simulink model "EMD_model_3"  (R2018b)
settings: Solver=ode45  StartTime=0  StopTime=setStopTime  FixedStep=0.0005  RelTol=1e-3  EnableMultiTasking=on
model workspace (MAT data in the model file):
  Body = timeseries
  Body.Name = 'unnamed'
  Body.DataInfo = tsdata.datametadata
  Body.DataInfo.Interpolation = tsdata.interpolation
  Body.DataInfo.Interpolation.Fhandle : function handle (value not decoded)
  Body.DataInfo.Interpolation.Name = 'linear'
  Body.TimeInfo = tsdata.timemetadata
  Body.TimeInfo.Length = 1
  Body.TimeInfo.DuplicateTimes = 0
  Body.TimeInfo.Time_ = 0
  Body.TimeInfo.Initialized = 1
  Body.QualityInfo = tsdata.qualmetadata
  Body.Data_ = 0
  Head = timeseries
  Head.Name = 'unnamed'
  Head.DataInfo = tsdata.datametadata
  Head.DataInfo.Interpolation = tsdata.interpolation
  Head.DataInfo.Interpolation.Fhandle : function handle (value not decoded)
  Head.DataInfo.Interpolation.Name = 'linear'
  Head.TimeInfo = tsdata.timemetadata
  Head.TimeInfo.Length = 1
  Head.TimeInfo.DuplicateTimes = 0
  Head.TimeInfo.Time_ = 0
  Head.TimeInfo.Initialized = 1
  Head.QualityInfo = tsdata.qualmetadata
  Head.Data_ = 0
  Stimulus = timeseries
  Stimulus.Name = 'unnamed'
  Stimulus.DataInfo = tsdata.datametadata
  Stimulus.DataInfo.Interpolation = tsdata.interpolation
  Stimulus.DataInfo.Interpolation.Fhandle : function handle (value not decoded)
  Stimulus.DataInfo.Interpolation.Name = 'linear'
  Stimulus.TimeInfo = tsdata.timemetadata
  Stimulus.TimeInfo.Length = 1002
  Stimulus.TimeInfo.DuplicateTimes = 0
  Stimulus.TimeInfo.Time_ = [0 1 1.001 1.002 1.003 1.004 1.005 1.006 1.007 1.008 1.009 1.01 ... (1002 elements, 1002x1)]
  Stimulus.TimeInfo.Initialized = 1
  Stimulus.QualityInfo = tsdata.qualmetadata
  Stimulus.Data_ = [0 0 0.000504970946371 0.00100994189274 0.00151491283911 0.00201988378549 0.00252485473186 0.00302982567823 0.0035347966246 0.00403976757097 0.00454473851734 0.00504970946371 ... (1002 elements, 1002x1)]
  bodyAmp = 0
  bodyPhase = 0
  freq = 628.318530718
  headAmp = 0
  headPhase = 0
  high_delay = 0
  imageData = [0.0103288684164 0.0102822233939 0.0102126505282 0.0101206184381 0.0100067437275 0.00987178410641 0.00971662999494 0.00954229474258 0.00934990361191 0.00914068169451 0.00891594094035 0.0086770664925 0.0084255025256 0.00816273778989 0.00789029106167 0.00760969669731 0.00732249048001 0.00703019593824 0.0067343113009 0.00643629723877 0.00613756552338 0.00583946871534 0.00554329097296 0.00525024005097 0.00496144053728 0.0046779283543 0.00440064653061 0.00413044222873 0.00386806499661 0.0036141661931 0.00336929952316 0.00313392260524 0.00290839948268 0.00269300398237 0.00248792381768 0.00229326532855 0.00210905874991 0.0019352638995 0.00177177617837 0.00161843278107 0.00147501901756 0.00134127465545 0.00121690019877 0.00110156302754 0.000994903331533 0.0015437397287 0.00152917487879 0.00152917487879 0.0015437397287 0.000994903331533 0.00110156302754 0.00121690019877 0.00134127465545 0.00147501901756 0.00161843278107 0.00177177617837 0.0019352638995 0.00210905874991 0.00229326532855 0.00248792381768 0.00269300398237 0.00290839948268 0.00313392260524 0.00336929952316 0.0036141661931 0.00386806499661 0.00413044222873 0.00440064653061 0.0046779283543 0.00496144053728 0.00525024005097 0.00554329097296 0.00583946871534 0.00613756552338 0.00643629723877 0.0067343113009 0.00703019593824 0.00732249048001 0.00760969669731 0.00789029106167 0.00816273778989 0.0084255025256 0.0086770664925 0.00891594094035 0.00914068169451 0.00934990361191 0.00954229474258 0.00971662999494 0.00987178410641 0.0100067437275 0.0101206184381 0.0102126505282 0.0102822233939 0.0103288684164 0.0103522702192 0.0103522702192]
  low_delay = 0.03
  outputTimeList = [1 1.001 1.002 1.003 1.004 1.005 1.006 1.007 1.008 1.009 1.01 1.011 ... (1001 elements, 1x1001)]
  photo_a = 1
  photo_b = 1
  setStartTime = 5.68986602902
  setStopTime = 2
  stimAmp = 15
  temporalFilt = 0.035
  timeConstant = 0.06
libraries: visionsources x1
settings Model: SimulationMode=accelerator  Creator=Shane  LastModifiedBy=boc5244
settings DataIOCC: SaveFormat=Array  ReturnWorkspaceOutputs=on  OutputOption=SpecifiedOutputTimes  OutputTimes=outputTimeList
settings OptimizationCC: ExpressionDepthLimit=2147483647  EfficientMapNaN2IntZero=off  SimCompilerOptimization=on
settings DebuggingCC: UnderspecifiedInitializationDetection=Classic  MergeDetectMultiDrivingBlocksExec=none  FcnCallInpInsideContextMsg=warning  StateNameClashWarn=warning  SFUnexpectedBacktrackingDiag=warning  SFNoUnconditionalDefaultTransitionDiag=warning  SFExecutionAtInitializationDiag=none
settings HardwareCC: ProdBitPerPointer=32  ProdBitPerSizeT=32  ProdBitPerPtrDiffT=32  ProdLargestAtomicFloat=None  ProdIntDivRoundTo=Undefined  ProdEndianess=Unspecified  ProdWordSize=32  ProdHWDeviceType=32-bit Generic  TargetBitPerPointer=64  TargetBitPerSizeT=64  TargetBitPerPtrDiffT=64  TargetLongLongMode=on  TargetIntDivRoundTo=Zero  TargetEndianess=LittleEndian  TargetWordSize=64  TargetHWDeviceType=MATLAB Host  ProdEqTarget=off
settings ModelReferenceCC: PropagateSignalLabelsOutOfModel=off
settings SFSimCC: SimUseLocalCustomCode=off
settings RTWCC: SystemTargetFile=accel.tlc  TemplateMakefile=accel_default_tmf  RTWVerbose=off
settings CodeAppCC: MaxIdLength=128
settings STFCustomTargetCC: ConcurrentExecutionCompliant=on  MATLABClassNameForMDSCustomization=Simulink.SoftwareTarget.TargetSpecificTriggerConfigurationBase  GRTInterface=on  SystemTargetFile=accel.tlc
settings ConfigComp: CovMetricSettings=dw  CovHtmlReporting=on  CovSaveCumulativeToWorkspaceVar=on  CovSaveSingleToWorkspaceVar=on  CovExternalEMLEnable=off

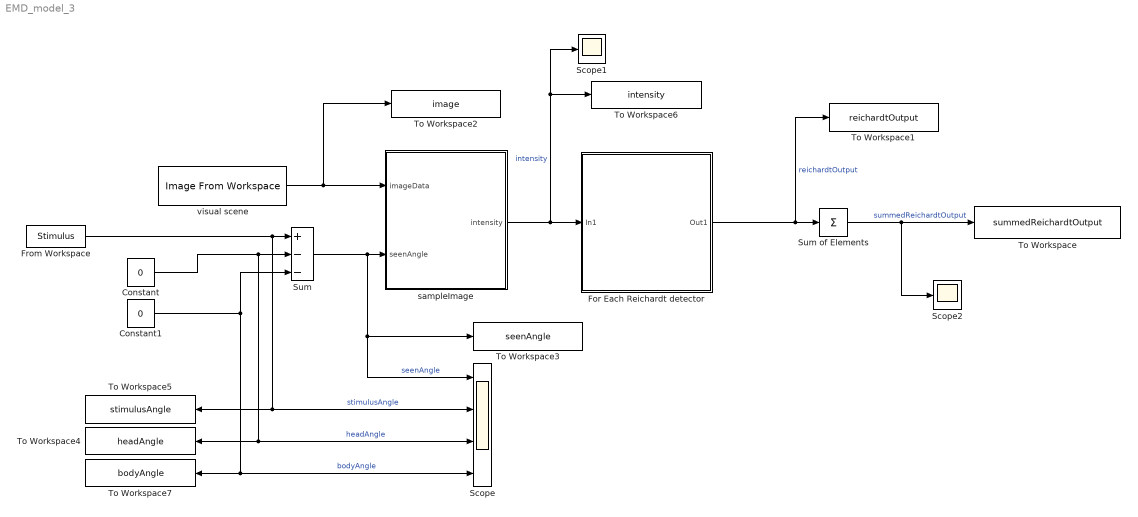
== system EMD_model_3 ==
  Constant : Constant  Value=0
  Constant1 : Constant  Value=0
  For Each Reichardt detector : Subsystem  TreatAsAtomicUnit=on
  From Workspace : FromWorkspace  VariableName=Stimulus  SampleTime=0  OutputAfterFinalValue=Setting to zero
  Scope : Scope  NumInputPorts=4
  Scope1 : Scope
  Scope2 : Scope
  Sum : Sum  Inputs=+--
  Sum of Elements : Sum  Inputs=+
  To Workspace : ToWorkspace  VariableName=summedReichardtOutput  SaveFormat=Timeseries  SampleTime=-1
  To Workspace1 : ToWorkspace  VariableName=reichardtOutput  SaveFormat=Timeseries  SampleTime=-1
  To Workspace2 : ToWorkspace  VariableName=image  SaveFormat=Timeseries  SampleTime=-1
  To Workspace3 : ToWorkspace  VariableName=seenAngle  SaveFormat=Timeseries  SampleTime=-1
  To Workspace4 : ToWorkspace  VariableName=headAngle  SaveFormat=Timeseries  SampleTime=-1
  To Workspace5 : ToWorkspace  VariableName=stimulusAngle  SaveFormat=Timeseries  SampleTime=-1
  To Workspace6 : ToWorkspace  VariableName=intensity  SaveFormat=Timeseries  SampleTime=-1
  To Workspace7 : ToWorkspace  VariableName=bodyAngle  SaveFormat=Timeseries  SampleTime=-1
  sampleImage : MATLAB Function  TreatAsAtomicUnit=on
  visual scene : visionsources/Image From Workspace  Tag=vipblks_nd  ImageValue=imageData  Ts=inf  imagePorts=One multidimensional signal  OutPortLabels=R|G|B  ImageDataType=double  Signed=on  WordLength=16  sdImageDataType=sfix(16)  FractionLengthMode=User-defined  FractionLength=15
      settings: SourceProductName=Computer Vision Toolbox  SourceProductBaseCode=VP
  wires:
  For Each Reichardt detector/1(Out1) -> To Workspace1/1, Sum of Elements/1  "reichardtOutput"
  Sum of Elements/1 -> Scope2/1, To Workspace/1  "summedReichardtOutput"
  sampleImage/1(intensity) -> Scope1/1, To Workspace6/1, For Each Reichardt detector/1(In1)  "intensity"
  visual scene/1 -> To Workspace2/1, sampleImage/1(imageData)
  From Workspace/1 -> To Workspace5/1, Scope/2, Sum/1  "stimulusAngle"
  Constant/1 -> To Workspace4/1, Scope/3, Sum/2  "headAngle"
  Sum/1 -> Scope/1, To Workspace3/1, sampleImage/2(seenAngle)  "seenAngle"
  Constant1/1 -> Sum/3, To Workspace7/1, Scope/4  "bodyAngle"

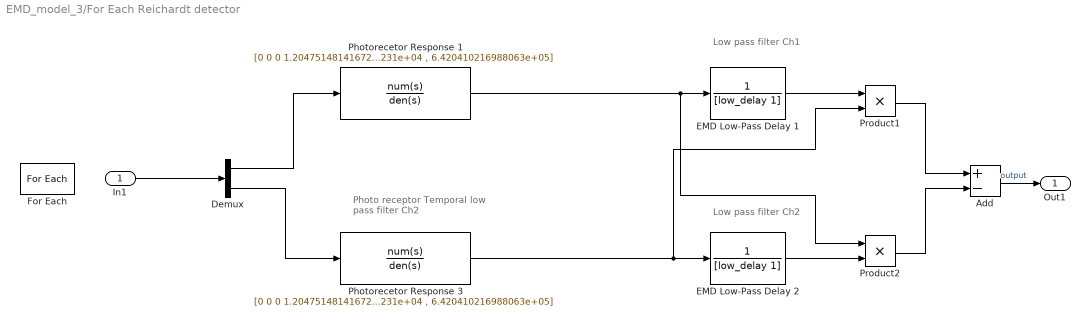
== system EMD_model_3/For Each Reichardt detector ==
  note: Photo receptor
      | Temporal low pass filter
      | Ch2
  note: Low pass filter
      | Ch1
  note: Low pass filter
      | Ch2
  In1 : Inport  Partition=on  PartitionDimension=1  PartitionWidth=1  PartitionOffset=0
  Add : Sum  Inputs=+-
  Demux : Demux  Outputs=2
  EMD Low-Pass Delay 1 : TransferFcn  Denominator=[low_delay 1]
  EMD Low-Pass Delay 2 : TransferFcn  Denominator=[low_delay 1]
  For Each : ForEach  DisableCoverage=on  IndexMode=One-based
  Photorecetor Response 1 : TransferFcn  Numerator=[0 0 0 1.204751481416720e+09]  Denominator=[1 , 2.807494939800572e+02 , 3.207046876121231e+04 , 6.420410216988063e+05]
  Photorecetor Response 3 : TransferFcn  Numerator=[0 0 0 1.204751481416720e+09]  Denominator=[1 , 2.807494939800572e+02 , 3.207046876121231e+04 , 6.420410216988063e+05]
  Product1 : Product  RndMeth=Zero
  Product2 : Product  RndMeth=Zero
  Out1 : Outport  ConcatenationDimension=1
  wires:
  EMD Low-Pass Delay 1/1 -> Product1/1
  Product1/1 -> Add/1
  Product2/1 -> Add/2
  EMD Low-Pass Delay 2/1 -> Product2/2
  Add/1 -> Out1/1  "output"
  In1/1 -> Demux/1
  Demux/1 -> Photorecetor Response 1/1
  Demux/2 -> Photorecetor Response 3/1
  Photorecetor Response 1/1 -> EMD Low-Pass Delay 1/1, Product2/1
  Photorecetor Response 3/1 -> EMD Low-Pass Delay 2/1, Product1/2

== matlab function EMD_model_3/sampleImage ==
  data: imageData input; intensity output double size=360,2; seenAngle input
function intensity = fcn(imageData,seenAngle)
%#codegen

imageWidth = length(imageData);

% Subsample with resolution of compound eye
sampleCoord = 0:359;
sampleCoord = sampleCoord + seenAngle;
sampleCoord = mod(sampleCoord,360);
temp        = interp1(linspace(0,360,imageWidth),imageData,sampleCoord);

% Create output signals
intensity = [temp(:), circshift(temp(:),-1)];
